simulink model "gm_Lab2_2"  (R2022a)
settings: Solver=VariableStepAuto  StartTime=0.0  StopTime=10.0  RelTol=1e-3
settings Model: Creator=Dubov  LastModifiedBy=Dubov
settings OptimizationCC: BlockReduction=off  ConditionallyExecuteInputs=off
settings DebuggingCC: InheritedTsInSrcMsg=none

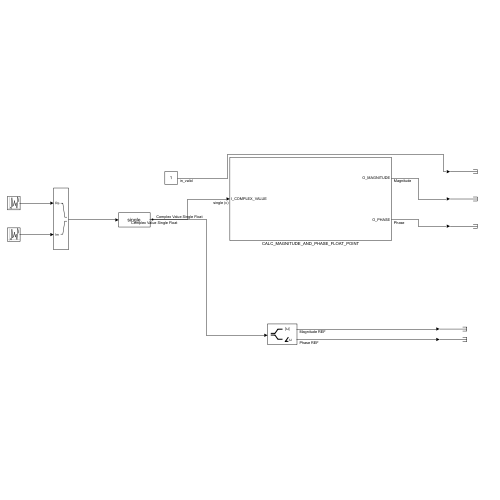
[thumbnail: Simulink's stored preview of the top-level diagram]
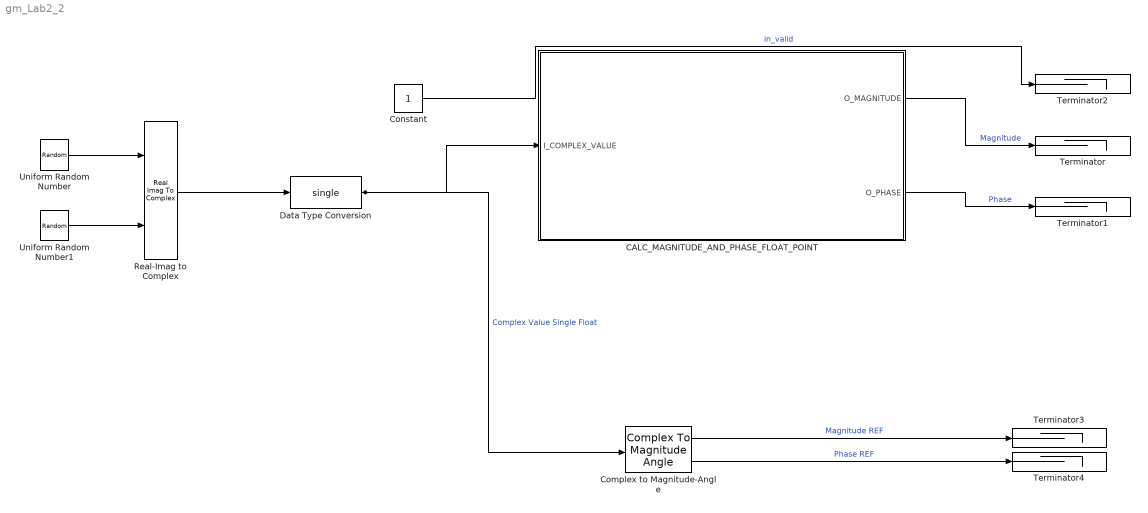
== system gm_Lab2_2 ==
  CALC_MAGNITUDE_AND_PHASE_FLOAT_POINT : Subsystem
  Complex to Magnitude-Angle : ComplexToMagnitudeAngle
  Constant : Constant  OutDataTypeStr=boolean
  Data Type Conversion : DataTypeConversion  OutDataTypeStr=single  RndMeth=Round  SaturateOnIntegerOverflow=off
  Real-Imag to Complex : RealImagToComplex
  Terminator{,1..4} (5 alike) : Terminator
  Uniform Random Number : UniformRandomNumber  Minimum=0  Maximum=2^(20)-1  Seed=20  SampleTime=1
  Uniform Random Number1 : UniformRandomNumber  Minimum=0  Maximum=2^(20)-1  Seed=21  SampleTime=1
  wires:
  Constant/1 -> Terminator2/1  "in_valid"
  Complex to Magnitude-Angle/2 -> Terminator4/1  "Phase REF"
  Uniform Random Number/1 -> Real-Imag to Complex/1
  Uniform Random Number1/1 -> Real-Imag to Complex/2
  Complex to Magnitude-Angle/1 -> Terminator3/1  "Magnitude REF"
  Real-Imag to Complex/1 -> Data Type Conversion/1
  CALC_MAGNITUDE_AND_PHASE_FLOAT_POINT/1(O_MAGNITUDE) -> Terminator/1  "Magnitude"
  CALC_MAGNITUDE_AND_PHASE_FLOAT_POINT/2(O_PHASE) -> Terminator1/1  "Phase"
  Data Type Conversion/1 -> Complex to Magnitude-Angle/1, CALC_MAGNITUDE_AND_PHASE_FLOAT_POINT/1(I_COMPLEX_VALUE)  "Complex Value Single Float"

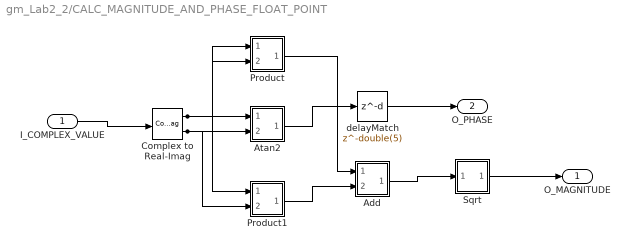
== system gm_Lab2_2/CALC_MAGNITUDE_AND_PHASE_FLOAT_POINT ==
  I_COMPLEX_VALUE : Inport  OutDataTypeStr=single  PortDimensions=1  SampleTime=1
      settings: SignalType=complex
  Add : Subsystem
      mask Display: disp('NFP\nadd');
  Atan2 : Subsystem
      mask Display: disp('NFP\ntrig3');
  Complex to Real-Imag : ComplexToRealImag  SampleTime=1
  Product : Subsystem
      mask Display: disp('NFP\nmul');
  Product1 : Subsystem
      mask Display: disp('NFP\nmul');
  Sqrt : Subsystem
      mask Display: disp('NFP\nsqrt');
  delayMatch : Delay  DelayLength=double(5)  InitialCondition=0  SampleTime=1
  O_MAGNITUDE : Outport  SampleTime=1
  O_PHASE : Outport  Port=2  SampleTime=1
  wires:
  I_COMPLEX_VALUE/1 -> Complex to Real-Imag/1
  delayMatch/1 -> O_PHASE/1
  Complex to Real-Imag/1 -> Product/2(In2), Product/1(In1), Atan2/2(In2)
  Complex to Real-Imag/2 -> Product1/2(In2), Product1/1(In1), Atan2/1(In1)
  Add/1(Out1) -> Sqrt/1(In1)
  Atan2/1(Out1) -> delayMatch/1
  Product/1(Out1) -> Add/1(In1)
  Product1/1(Out1) -> Add/2(In2)
  Sqrt/1(Out1) -> O_MAGNITUDE/1

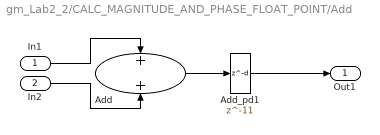
== system gm_Lab2_2/CALC_MAGNITUDE_AND_PHASE_FLOAT_POINT/Add ==
  In1 : Inport
  In2 : Inport  Port=2
  Add : Sum  OutDataTypeStr=single  SampleTime=1
  Add_pd1 : Delay  DelayLength=11
  Out1 : Outport
  wires:
  In1/1 -> Add/1
  In2/1 -> Add/2
  Add/1 -> Add_pd1/1
  Add_pd1/1 -> Out1/1

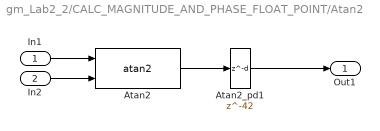
== system gm_Lab2_2/CALC_MAGNITUDE_AND_PHASE_FLOAT_POINT/Atan2 ==
  In1 : Inport
  In2 : Inport  Port=2
  Atan2 : Trigonometry  Operator=atan2  SampleTime=1
  Atan2_pd1 : Delay  DelayLength=42
  Out1 : Outport
  wires:
  In1/1 -> Atan2/1
  In2/1 -> Atan2/2
  Atan2/1 -> Atan2_pd1/1
  Atan2_pd1/1 -> Out1/1

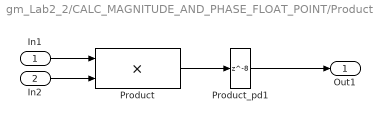
== system gm_Lab2_2/CALC_MAGNITUDE_AND_PHASE_FLOAT_POINT/Product ==
  In1 : Inport
  In2 : Inport  Port=2
  Product : Product  Inputs=**  OutDataTypeStr=single  SampleTime=1
  Product_pd1 : Delay  DelayLength=8
  Out1 : Outport
  wires:
  In1/1 -> Product/1
  In2/1 -> Product/2
  Product/1 -> Product_pd1/1
  Product_pd1/1 -> Out1/1

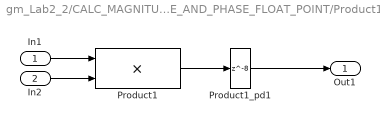
== system gm_Lab2_2/CALC_MAGNITUDE_AND_PHASE_FLOAT_POINT/Product1 ==
  In1 : Inport
  In2 : Inport  Port=2
  Product1 : Product  Inputs=**  OutDataTypeStr=single  SampleTime=1
  Product1_pd1 : Delay  DelayLength=8
  Out1 : Outport
  wires:
  In1/1 -> Product1/1
  In2/1 -> Product1/2
  Product1/1 -> Product1_pd1/1
  Product1_pd1/1 -> Out1/1

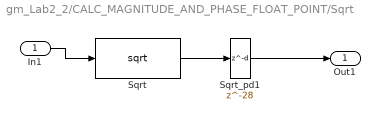
== system gm_Lab2_2/CALC_MAGNITUDE_AND_PHASE_FLOAT_POINT/Sqrt ==
  In1 : Inport
  Sqrt : Sqrt  SampleTime=1
  Sqrt_pd1 : Delay  DelayLength=28
  Out1 : Outport
  wires:
  In1/1 -> Sqrt/1
  Sqrt/1 -> Sqrt_pd1/1
  Sqrt_pd1/1 -> Out1/1
